simulink model "Part1B"  (R2025b)
settings: Solver=VariableStepAuto  StartTime=0.0  StopTime=10.0  RelTol=1e-3
settings Model: Creator=hashaamzafar  LastModifiedBy=hashaamzafar

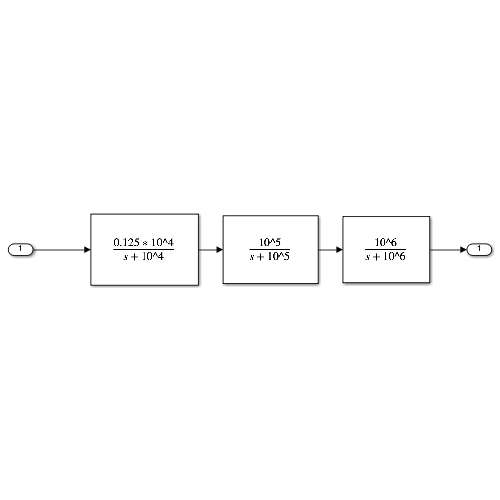
[thumbnail: Simulink's stored preview of the top-level diagram]
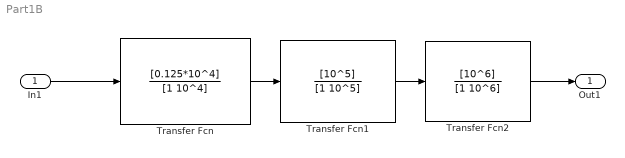
== system Part1B ==
  In1 : Inport
  Transfer Fcn : TransferFcn  Numerator=[0.125*10^4]  Denominator=[1 10^4]
  Transfer Fcn1 : TransferFcn  Numerator=[10^5]  Denominator=[1 10^5]
  Transfer Fcn2 : TransferFcn  Numerator=[10^6]  Denominator=[1 10^6]
  Out1 : Outport
  wires:
  Transfer Fcn/1 -> Transfer Fcn1/1
  Transfer Fcn1/1 -> Transfer Fcn2/1
  In1/1 -> Transfer Fcn/1
  Transfer Fcn2/1 -> Out1/1
